simulink model "SIMULINK"  (R2024b)
settings: Solver=VariableStepAuto  StartTime=0.0  StopTime=100  RelTol=1e-3
values from neighbouring files (symbols this model uses):
  A = [ 0        1           0           0 ... (first row only)    [Passive_Simulink.m]    (also in Passive_sus.m; Passive_sus_ISO.m; Roadsimulation.m = sqrt(2*Gd*dn); animation_gui.m = [0, 1, 0, 0)
  Bu = [0; 1/m1; 0; -1/m2]    [Passive_Simulink.m]    (also in Passive_sus.m; Passive_sus_ISO.m; animation_gui.m; lqr_pcode.m)
  Bw = [0; 0; 0;  k2/m2]    [Passive_Simulink.m]    (also in Passive_sus.m = [0; 0; 0; k2/m2]; Passive_sus_ISO.m = [0; 0; 0; k2/m2]; animation_gui.m = [0; 0; 0; k2/m2]; lqr_pcode.m = [0; 0; 0; k2/m2])
  C_y1 = [1 0 -1 0]    [Passive_Simulink.m]
  D_y1 = [0 0]    [Passive_Simulink.m]
  K = place(A, Bu, p_des)    [Passive_Simulink.m]    (also in Passive_sus.m; Passive_sus_ISO.m)
  Nw = -(C_y1*(Acl\Bw)) / (C_y1*(Acl\Bu))    [Passive_Simulink.m]    (also in Passive_sus.m = -(C*(Acl\Bw)) / (C*(Acl\Bu)); Passive_sus_ISO.m = -(C*(Acl\Bw)) / den; rampthenbump.m = -(C*(Acl\Bw)) / (C*(Acl\Bu)))
settings Model: Creator=every  LastModifiedBy=every

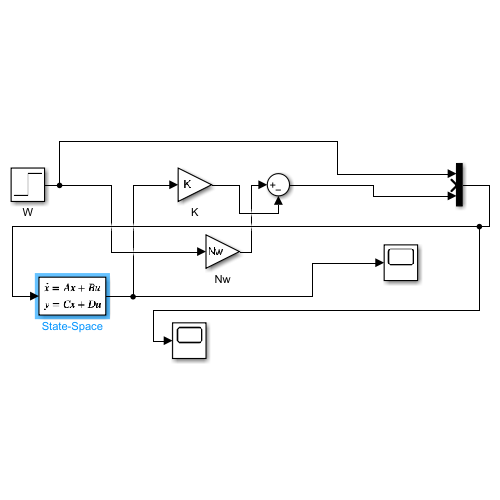
[thumbnail: Simulink's stored preview of the top-level diagram]
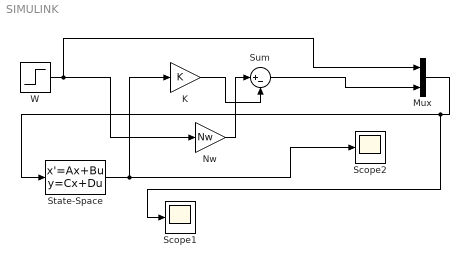
== system SIMULINK ==
  K : Gain  Gain=K
  Mux : Mux  Inputs=3
  Nw : Gain  Gain=Nw
  Scope1 : Scope
  Scope2 : Scope
  State-Space : StateSpace  A=A  B=[Bu Bw]  C=C_y1  D=D_y1  InitialCondition=0  AllowTunableDMatrix=on
  Sum : Sum  Inputs=|+-
  W : Step  Time=0  After=.1  SampleTime=0
  wires:
  W/1 -> Mux/1, Nw/1
  State-Space/1 -> K/1, Scope2/1
  Sum/1 -> Mux/3
  Mux/1 -> State-Space/1, Scope1/1
  K/1 -> Sum/2
  Nw/1 -> Sum/1
